simulink model "Inverse_Dynamic_Control"  (R2023b)
settings: Solver=FixedStepAuto  StartTime=0.0  StopTime=10.0  FixedStep=sampleTime  RelTol=1e-3
undefined symbols (not defined in the file): initial, initialPos, robot
libraries: robotmaniplib x5, robotcorelib x2
settings Model: Creator=jake9  LastModifiedBy=jake9

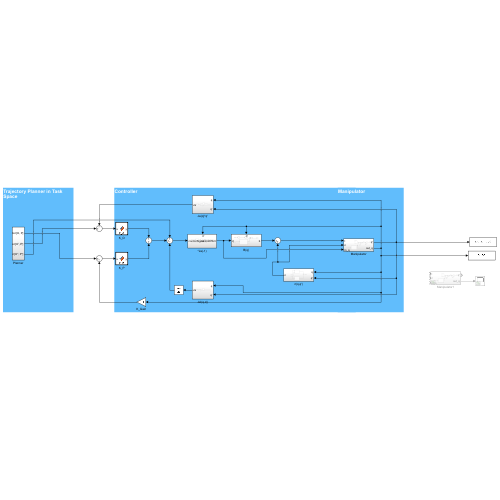
[thumbnail: Simulink's stored preview of the top-level diagram]
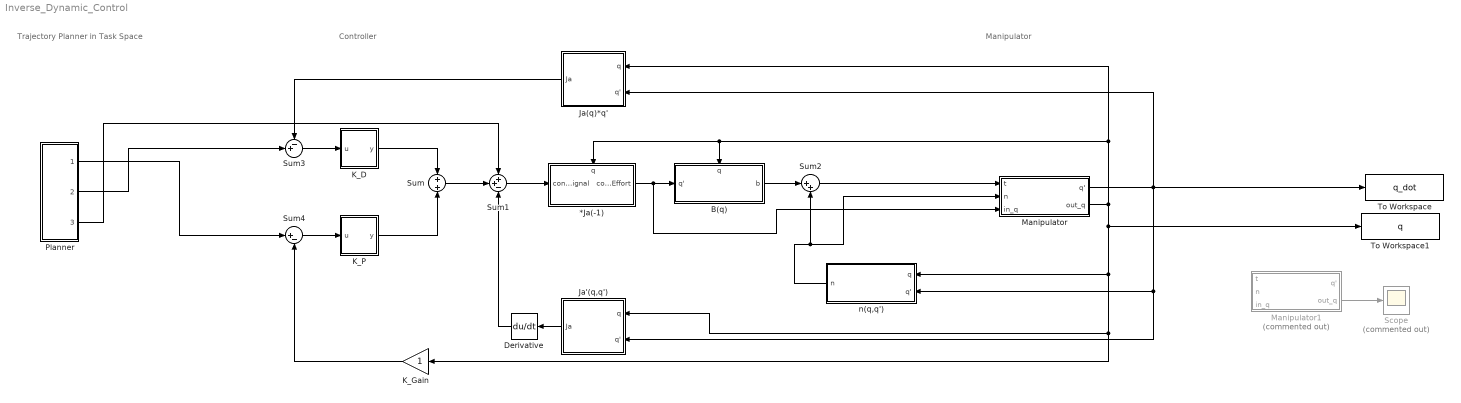
== system Inverse_Dynamic_Control ==
  note: Manipulator
  note: Trajectory Planner in Task Space
  note: Controller
  *Ja(-1) : Subsystem
      settings: PortSchema="{\"entries\":[{\"content\":{\"sides\":[{\"content\":{\"connectorIds\":[\"In1\"]},\"type\":\"ConnectorPlacement.EquallySpacedRectSide\",\"uuid\":\"6181597d-d95a-4c94-8b0a-1b126e10fdbf\"},{\"content\":{\"connectorIds\":[\"Out1\"],\"side\":\"RIGHT\"},\"type\":\"ConnectorPlacement.EquallySpacedRectSide\",\"uuid\":\"10cd4102-ac71-40d2-b2d5-351b2662a651\"},{\"content\":{\"connectorIds\":[\"In2\"],\"side\":\"TOP\"},\"type\":\"ConnectorPlacement.EquallySpacedRectSide\",\"uuid\":\"51fc8434-6bfd-4c46-b058-3c914862beda\"}]},\"type\":\"ConnectorPlacement.EquallySpacedConnector\",\"uuid\":\"e6979264-e48a-4d32-b7c0-5cbd3e80f60c\"}],\"packageUris\":[\"http://schema.mathworks.com/mf0/Connector/R2020b\"],\"version\":\"1.0\"}"
  B(q) : Subsystem
      settings: PortSchema="{\"entries\":[{\"content\":{\"sides\":[{\"content\":{\"connectorIds\":[\"In1\"]},\"type\":\"ConnectorPlacement.EquallySpacedRectSide\",\"uuid\":\"6181597d-d95a-4c94-8b0a-1b126e10fdbf\"},{\"content\":{\"connectorIds\":[\"Out1\"],\"side\":\"RIGHT\"},\"type\":\"ConnectorPlacement.EquallySpacedRectSide\",\"uuid\":\"10cd4102-ac71-40d2-b2d5-351b2662a651\"},{\"content\":{\"connectorIds\":[\"In2\"],\"side\":\"TOP\"},\"type\":\"ConnectorPlacement.EquallySpacedRectSide\",\"uuid\":\"51fc8434-6bfd-4c46-b058-3c914862beda\"}]},\"type\":\"ConnectorPlacement.EquallySpacedConnector\",\"uuid\":\"e6979264-e48a-4d32-b7c0-5cbd3e80f60c\"}],\"packageUris\":[\"http://schema.mathworks.com/mf0/Connector/R2020b\"],\"version\":\"1.0\"}"
  Derivative : Derivative
  Ja'(q,q') : Subsystem
  Ja(q)*q' : Subsystem
  K_D : MATLAB Function  TreatAsAtomicUnit=on
  K_Gain : Gain
  K_P : MATLAB Function  TreatAsAtomicUnit=on
  Manipulator : Subsystem
  Manipulator1 : Subsystem  Commented=on
  Planner : Subsystem
  Scope : Scope  Commented=on
  Sum : Sum  Inputs=+|+
  Sum1 : Sum  Inputs=++-
  Sum2 : Sum  Inputs=|++
  Sum3 : Sum  Inputs=-+|
  Sum4 : Sum  Inputs=|+-
  To Workspace : ToWorkspace  VariableName=q_dot  SampleTime=-1
  To Workspace1 : ToWorkspace  VariableName=q  SampleTime=-1
  n(q,q') : Subsystem
  wires:
  K_D/1(y) -> Sum/1
  K_P/1(y) -> Sum/2
  Sum/1 -> Sum1/2
  Sum1/1 -> *Ja(-1)/1(controlSignal)
  *Ja(-1)/1(controlEffort) -> Manipulator/3(in_q), B(q)/1(q')
  B(q)/1(b) -> Sum2/1
  Sum3/1 -> K_D/1(u)
  Sum4/1 -> K_P/1(u)
  K_Gain/1 -> Sum4/2
  n(q,q')/1(n) -> Manipulator/2(n), Sum2/2
  Sum2/1 -> Manipulator/1(t)
  Manipulator/2(out_q) -> Ja(q)*q'/1(q), *Ja(-1)/2(q), B(q)/2(q), To Workspace1/1, n(q,q')/1(q), Ja'(q,q')/1(q), K_Gain/1
  Manipulator/1(q') -> n(q,q')/2(q'), Ja'(q,q')/2(q'), Ja(q)*q'/2(q'), To Workspace/1
  Ja(q)*q'/1(Ja) -> Sum3/1
  Ja'(q,q')/1(Ja) -> Derivative/1
  Derivative/1 -> Sum1/3
  Planner/1("Out [O, P]") -> Sum4/1
  Planner/2("Out [O', P']") -> Sum3/2
  Planner/3("Out [O'', P'']") -> Sum1/1
  Manipulator1/2(out_q) -> Scope/1

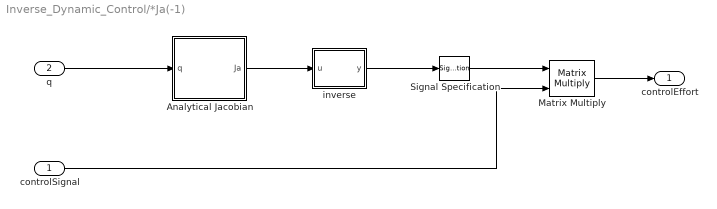
== system Inverse_Dynamic_Control/*Ja(-1) ==
  controlSignal : Inport
  q : Inport  Port=2
  Analytical Jacobian : Subsystem
  Matrix Multiply : Product  Multiplication=Matrix(*)
  Signal Specification : SignalSpecification  Dimensions=[6,6]
  inverse : MATLAB Function  TreatAsAtomicUnit=on
  controlEffort : Outport
  wires:
  q/1 -> Analytical Jacobian/1(q)
  controlSignal/1 -> Matrix Multiply/2
  inverse/1(y) -> Signal Specification/1
  Analytical Jacobian/1(Ja) -> inverse/1(u)
  Matrix Multiply/1 -> controlEffort/1
  Signal Specification/1 -> Matrix Multiply/1

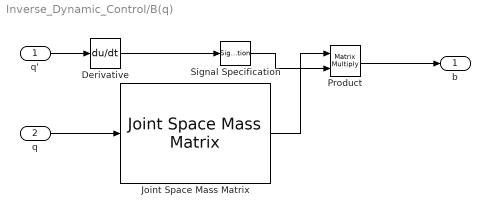
== system Inverse_Dynamic_Control/B(q) ==
  q' : Inport
  q : Inport  Port=2
  Derivative : Derivative
  Joint Space Mass Matrix : robotmaniplib/Joint Space Mass Matrix  RigidBodyTree=robot  SimulateUsing=Interpreted execution
  Product : Product  Multiplication=Matrix(*)
  Signal Specification : SignalSpecification  Dimensions=[6,1]
  b : Outport
  wires:
  q'/1 -> Derivative/1
  q/1 -> Joint Space Mass Matrix/1
  Product/1 -> b/1
  Derivative/1 -> Signal Specification/1
  Joint Space Mass Matrix/1 -> Product/1
  Signal Specification/1 -> Product/2

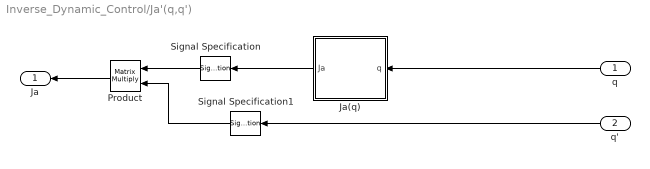
== system Inverse_Dynamic_Control/Ja'(q,q') ==
  q : Inport
  q' : Inport  Port=2
  Ja(q) : Subsystem
  Product : Product  Multiplication=Matrix(*)
  Signal Specification : SignalSpecification  Dimensions=[6,6]
  Signal Specification1 : SignalSpecification  Dimensions=[6,1]
  Ja : Outport
  wires:
  q/1 -> Ja(q)/1(q)
  q'/1 -> Signal Specification1/1
  Product/1 -> Ja/1
  Ja(q)/1(Ja) -> Signal Specification/1
  Signal Specification/1 -> Product/1
  Signal Specification1/1 -> Product/2

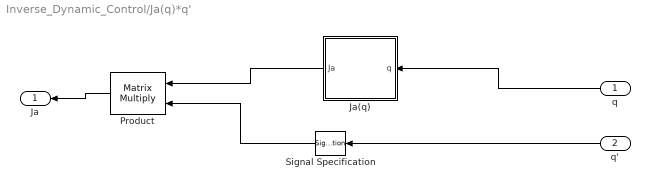
== system Inverse_Dynamic_Control/Ja(q)*q' ==
  q : Inport
  q' : Inport  Port=2
  Ja(q) : Subsystem
  Product : Product  Multiplication=Matrix(*)
  Signal Specification : SignalSpecification  Dimensions=[6,1]
  Ja : Outport
  wires:
  q/1 -> Ja(q)/1(q)
  Product/1 -> Ja/1
  Ja(q)/1(Ja) -> Product/1
  q'/1 -> Signal Specification/1
  Signal Specification/1 -> Product/2

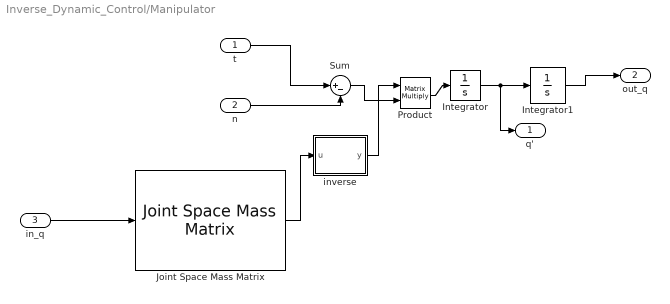
== system Inverse_Dynamic_Control/Manipulator ==
  t : Inport
  n : Inport  Port=2
  in_q : Inport  Port=3
  Integrator : Integrator  InitialCondition=initial
  Integrator1 : Integrator  InitialCondition=initialPos
  Joint Space Mass Matrix : robotmaniplib/Joint Space Mass Matrix  RigidBodyTree=robot  SimulateUsing=Interpreted execution
  Product : Product  Multiplication=Matrix(*)
  Sum : Sum  Inputs=|+-
  inverse : MATLAB Function  TreatAsAtomicUnit=on
  q' : Outport
  out_q : Outport  Port=2
  wires:
  Integrator/1 -> q'/1, Integrator1/1
  t/1 -> Sum/1
  n/1 -> Sum/2
  inverse/1(y) -> Product/1
  Sum/1 -> Product/2
  Product/1 -> Integrator/1
  Integrator1/1 -> out_q/1
  Joint Space Mass Matrix/1 -> inverse/1(u)
  in_q/1 -> Joint Space Mass Matrix/1

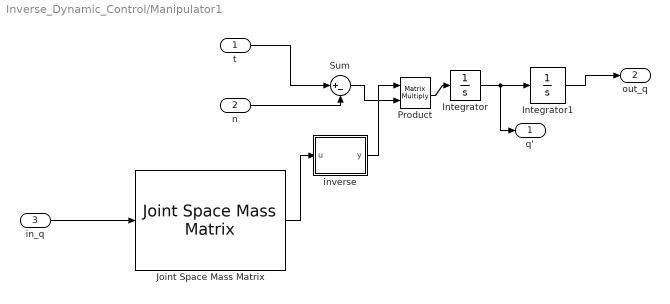
== system Inverse_Dynamic_Control/Manipulator1 ==
  t : Inport
  n : Inport  Port=2
  in_q : Inport  Port=3
  Integrator : Integrator  InitialCondition=initial
  Integrator1 : Integrator  InitialCondition=initialPos
  Joint Space Mass Matrix : robotmaniplib/Joint Space Mass Matrix  RigidBodyTree=robot  SimulateUsing=Interpreted execution
  Product : Product  Multiplication=Matrix(*)
  Sum : Sum  Inputs=|+-
  inverse : MATLAB Function  TreatAsAtomicUnit=on
  q' : Outport
  out_q : Outport  Port=2
  wires:
  Integrator/1 -> q'/1, Integrator1/1
  t/1 -> Sum/1
  n/1 -> Sum/2
  inverse/1(y) -> Product/1
  Sum/1 -> Product/2
  Product/1 -> Integrator/1
  Integrator1/1 -> out_q/1
  Joint Space Mass Matrix/1 -> inverse/1(u)
  in_q/1 -> Joint Space Mass Matrix/1

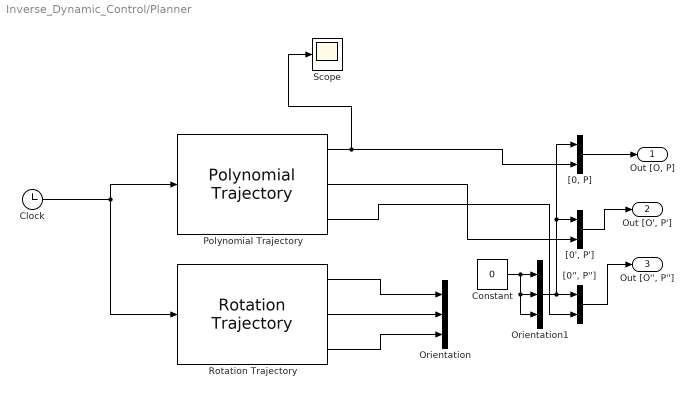
== system Inverse_Dynamic_Control/Planner ==
  Clock : Clock
  Constant : Constant  Value=0
  Orientation : Mux  Inputs=3
  Orientation1 : Mux  Inputs=3
  Polynomial Trajectory : robotcorelib/Polynomial Trajectory  WaypointSource=Internal  Waypoints=[1 1 1; 2 2 2; 3 3 3]'  TimePoints=[0, 4, 8]  TimeInterval=[ 1, 4 ]  Method=Cubic Polynomial  ParameterSource=Internal  VelocityBoundaryCondition=zeros( 3,3 )  AccelerationBoundaryCondition=zeros( 2, 5 )  SimulateUsing=Interpreted execution
  Rotation Trajectory : robotcorelib/Rotation Trajectory  WaypointFormat=Quaternion  WaypointSource=Internal  R0=[ 1, 0, 0, 0 ]'  RF=[ 0, 0, 1, 0 ]'  TimeInterval=[ 0, 8]  CustomTimeScaling=off  ParameterSource=Internal  TSTime=0:0.1:1  TimeScaling=[ 0:0.1:1; ones( 1, 11 ); zeros( 1, 11 ) ]  SimulateUsing=Interpreted execution
      settings: LibrarySourceBlock=robotutilslib/Rotation Trajectory
  Scope : Scope
  "[0'', P'']" : Mux  Inputs=2
  "[0', P']" : Mux  Inputs=2
  "[0, P]" : Mux  Inputs=2
  "Out [O, P]" : Outport
  "Out [O', P']" : Outport  Port=2
  "Out [O'', P'']" : Outport  Port=3
  wires:
  Clock/1 -> Rotation Trajectory/1, Polynomial Trajectory/1
  Polynomial Trajectory/1 -> "[0, P]"/2, Scope/1
  Polynomial Trajectory/2 -> "[0', P']"/2
  Polynomial Trajectory/3 -> "[0'', P'']"/2
  Rotation Trajectory/3 -> Orientation/3
  Rotation Trajectory/2 -> Orientation/2
  Rotation Trajectory/1 -> Orientation/1
  "[0, P]"/1 -> "Out [O, P]"/1
  Constant/1 -> Orientation1/3, Orientation1/2, Orientation1/1
  Orientation1/1 -> "[0'', P'']"/1, "[0', P']"/1, "[0, P]"/1
  "[0', P']"/1 -> "Out [O', P']"/1
  "[0'', P'']"/1 -> "Out [O'', P'']"/1

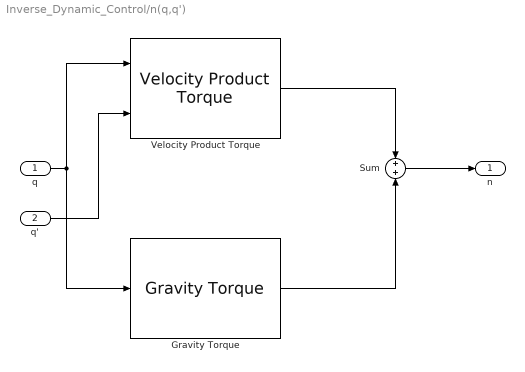
== system Inverse_Dynamic_Control/n(q,q') ==
  q : Inport
  q' : Inport  Port=2
  Gravity Torque : robotmaniplib/Gravity Torque  RigidBodyTree=robot  SimulateUsing=Interpreted execution
  Sum : Sum  Inputs=+|+
  Velocity Product Torque : robotmaniplib/Velocity Product Torque  RigidBodyTree=robot  SimulateUsing=Interpreted execution
  n : Outport
  wires:
  q/1 -> Gravity Torque/1, Velocity Product Torque/1
  q'/1 -> Velocity Product Torque/2
  Sum/1 -> n/1
  Gravity Torque/1 -> Sum/2
  Velocity Product Torque/1 -> Sum/1

== system Inverse_Dynamic_Control/*Ja(-1)/Analytical Jacobian ==
  note: Conversion of Jacobian, from Geometric to Analytical
      |
      | Matlab use the "Spatial Geometry" convenction, where the orientation in the first three rows instead of the last three rows. So we use:
      |
      | $J_{A}=\left[\begin{array}{cc} T^{-1} & 0 \\ 0 & I \end{array}\right]\left[\begin{array}{c} J_{O} \\ J_{P} \end{array}\right]=\left[\begin{array}{l} T^{-1} J_{O} \\ 0 \end{array}\right]+\left[\begin{array}{c} 0\\ J_{P} \end{array}\right] \quad \text {if } \,\, J=\left[\begin{array}{l} J_{O} \\ J_{P} \end{array}\right]$
      |
      | If orientation is in the last three rows (as in most of the text books) we would use instead:
      |
      | $J_{A}=\left[\begin{array}{cc} I & 0 \\ 0 & T^{-1} \end{array}\right]\left[\begin{array}{c} J_{P} \\ J_{O} \end{array}\right]=\left[\begin{array}{l} J_{P} \\ 0 \end{array}\right]+\left[\begin{array}{c} 0\\ T^{-1} J_{O} \end{array}\right] \quad \text { if } \,\, J=\left[\begin{array}{l} J_{P} \\ J_{O} \end{array}\right]$
  q : Inport
  Analytical from Geometric : MATLAB Function  TreatAsAtomicUnit=on
  Direct Kinematics : Subsystem
  Get Jacobian : Subsystem  mask(Get Jacobian){RigidBodyTree=robot, EndEffector=tool0, SimulateUsing=Code generation}
      mask prompts: RigidBodyTree "robotics:robotslmanip:blockmask:RigidBodyTreePrompt"; EndEffector "robotics:robotslmanip:blockmask:EndEffectorPrompt"; SimulateUsing "SystemBlock:MATLABSystem:SimulateUsing"
      mask help: robotics:robotslmanip:blockmask:GetJacobianDescription
      mask init:
      | try
      |    [TreeStruct, NumBodies, sysName] = robotics.slmanip.internal.block.RBTAlgorithmBlockMasks.updateMaskWorkSpaceVariables(gcb, RigidBodyTree);
      |    robotics.slmanip.internal.block.RBTAlgorithmBlockMasks.updateBlockInputDimensions(gcb, TreeStruct, 'Config');
      | catch ME
      |    TreeStruct = [];  NumBodies = [];   sysName = '???';
      |    throw(ME);
      | end
      | EndEffectorArray = robotics.slmanip.internal.block.RBTAlgorithmBlockMasks.updateBodyWSVar(gcb, RigidBodyTree, 'EndEffector');
      settings: LibrarySourceBlock=robotmaniplib/Get Jacobian
      mask Help: helpview(fullfile(docroot,'robotics','helptargets.map'), 'rstGetJacobian');
      mask TypeOptions SimulateUsing: MATLAB System/SimulateUsing
      mask DialogControl RigidBodyTree Prompt: Rigid body tree:
      mask DialogControl EndEffector Prompt: End effector:
      mask DialogControl ListControl Prompt: robotics:robotslmanip:blockmask:SelectBodyButtonPrompt
      mask DialogControl ListControl Callback: robotics.slmanip.internal.block.RBTAlgorithmBlockMasks.updateMaskBodyList(gcb, 'EndEffector');
      mask DialogControl SimulateUsing Prompt: Simulate using:
      mask DialogControl SimulateUsing Tooltip: SystemBlock:MATLABSystem:SimulateUsingDescription
      mask Display:
      | if (strcmp(sysName,'???'))
      | 	color('red');
      | else
      |     color('blue');
      | end
      | text(0.99, 0.99, sysName, 'horizontalAlignment', 'right', 'verticalAlignment','top');
      | 
      | color('black');
      | DescText = ['EE: ' get_param(gcb,'EndEffector')];
      | text(0.5, 0.05, DescText, 'horizontalAlignment', 'center', 'verticalAlignment','bottom');
      | 
      | port_label('input', 1, 'Config')
      | port_label('output', 1, 'Jacobian')
  Terminator : Terminator
  Ja : Outport
  wires:
  Direct Kinematics/1(orientation) -> Analytical from Geometric/2(angles)
  Direct Kinematics/2(position) -> Terminator/1
  Analytical from Geometric/1(Ja) -> Ja/1
  Get Jacobian/1(Jacobian) -> Analytical from Geometric/1(geomJ)
  q/1 -> Get Jacobian/1(Config), Direct Kinematics/1(q)

== system Inverse_Dynamic_Control/Ja'(q,q')/Ja(q) ==
  note: Conversion of Jacobian, from Geometric to Analytical
      |
      | Matlab use the "Spatial Geometry" convenction, where the orientation in the first three rows instead of the last three rows. So we use:
      |
      | $J_{A}=\left[\begin{array}{cc} T^{-1} & 0 \\ 0 & I \end{array}\right]\left[\begin{array}{c} J_{O} \\ J_{P} \end{array}\right]=\left[\begin{array}{l} T^{-1} J_{O} \\ 0 \end{array}\right]+\left[\begin{array}{c} 0\\ J_{P} \end{array}\right] \quad \text {if } \,\, J=\left[\begin{array}{l} J_{O} \\ J_{P} \end{array}\right]$
      |
      | If orientation is in the last three rows (as in most of the text books) we would use instead:
      |
      | $J_{A}=\left[\begin{array}{cc} I & 0 \\ 0 & T^{-1} \end{array}\right]\left[\begin{array}{c} J_{P} \\ J_{O} \end{array}\right]=\left[\begin{array}{l} J_{P} \\ 0 \end{array}\right]+\left[\begin{array}{c} 0\\ T^{-1} J_{O} \end{array}\right] \quad \text { if } \,\, J=\left[\begin{array}{l} J_{P} \\ J_{O} \end{array}\right]$
  q : Inport
  Analytical from Geometric : MATLAB Function  TreatAsAtomicUnit=on
  Direct Kinematics1 : Subsystem
  Get Jacobian : Subsystem  mask(Get Jacobian){RigidBodyTree=robot, EndEffector=tool0, SimulateUsing=Code generation}
      mask prompts: RigidBodyTree "robotics:robotslmanip:blockmask:RigidBodyTreePrompt"; EndEffector "robotics:robotslmanip:blockmask:EndEffectorPrompt"; SimulateUsing "SystemBlock:MATLABSystem:SimulateUsing"
      mask help: robotics:robotslmanip:blockmask:GetJacobianDescription
      mask init: same as Inverse_Dynamic_Control/*Ja(-1)/Analytical Jacobian/Get Jacobian
      settings: LibrarySourceBlock=robotmaniplib/Get Jacobian
      mask Help: helpview(fullfile(docroot,'robotics','helptargets.map'), 'rstGetJacobian');
      mask TypeOptions SimulateUsing: MATLAB System/SimulateUsing
      mask DialogControl RigidBodyTree Prompt: Rigid body tree:
      mask DialogControl EndEffector Prompt: End effector:
      mask DialogControl ListControl Prompt: robotics:robotslmanip:blockmask:SelectBodyButtonPrompt
      mask DialogControl ListControl Callback: robotics.slmanip.internal.block.RBTAlgorithmBlockMasks.updateMaskBodyList(gcb, 'EndEffector');
      mask DialogControl SimulateUsing Prompt: Simulate using:
      mask DialogControl SimulateUsing Tooltip: SystemBlock:MATLABSystem:SimulateUsingDescription
      mask Display:
      | if (strcmp(sysName,'???'))
      | 	color('red');
      | else
      |     color('blue');
      | end
      | text(0.99, 0.99, sysName, 'horizontalAlignment', 'right', 'verticalAlignment','top');
      | 
      | color('black');
      | DescText = ['EE: ' get_param(gcb,'EndEffector')];
      | text(0.5, 0.05, DescText, 'horizontalAlignment', 'center', 'verticalAlignment','bottom');
      | 
      | port_label('input', 1, 'Config')
      | port_label('output', 1, 'Jacobian')
  Terminator : Terminator
  Ja : Outport
  wires:
  Analytical from Geometric/1(Ja) -> Ja/1
  Get Jacobian/1(Jacobian) -> Analytical from Geometric/1(geomJ)
  q/1 -> Direct Kinematics1/1(q), Get Jacobian/1(Config)
  Direct Kinematics1/2(position) -> Terminator/1
  Direct Kinematics1/1(orientation) -> Analytical from Geometric/2(angles)

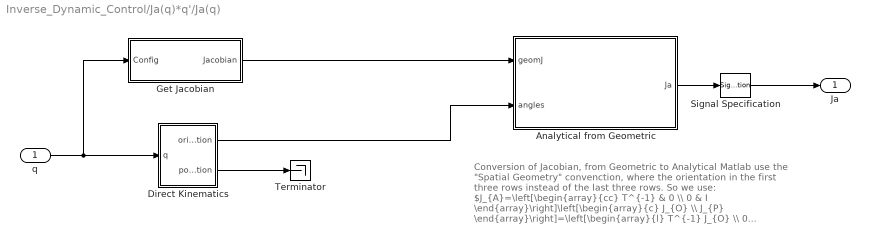
== system Inverse_Dynamic_Control/Ja(q)*q'/Ja(q) ==
  note: Conversion of Jacobian, from Geometric to Analytical
      |
      | Matlab use the "Spatial Geometry" convenction, where the orientation in the first three rows instead of the last three rows. So we use:
      |
      | $J_{A}=\left[\begin{array}{cc} T^{-1} & 0 \\ 0 & I \end{array}\right]\left[\begin{array}{c} J_{O} \\ J_{P} \end{array}\right]=\left[\begin{array}{l} T^{-1} J_{O} \\ 0 \end{array}\right]+\left[\begin{array}{c} 0\\ J_{P} \end{array}\right] \quad \text {if } \,\, J=\left[\begin{array}{l} J_{O} \\ J_{P} \end{array}\right]$
      |
      | If orientation is in the last three rows (as in most of the text books) we would use instead:
      |
      | $J_{A}=\left[\begin{array}{cc} I & 0 \\ 0 & T^{-1} \end{array}\right]\left[\begin{array}{c} J_{P} \\ J_{O} \end{array}\right]=\left[\begin{array}{l} J_{P} \\ 0 \end{array}\right]+\left[\begin{array}{c} 0\\ T^{-1} J_{O} \end{array}\right] \quad \text { if } \,\, J=\left[\begin{array}{l} J_{P} \\ J_{O} \end{array}\right]$
  q : Inport
  Analytical from Geometric : MATLAB Function  TreatAsAtomicUnit=on
  Direct Kinematics : Subsystem
  Get Jacobian : Subsystem  mask(Get Jacobian){RigidBodyTree=robot, EndEffector=tool0, SimulateUsing=Code generation}
      mask prompts: RigidBodyTree "robotics:robotslmanip:blockmask:RigidBodyTreePrompt"; EndEffector "robotics:robotslmanip:blockmask:EndEffectorPrompt"; SimulateUsing "SystemBlock:MATLABSystem:SimulateUsing"
      mask help: robotics:robotslmanip:blockmask:GetJacobianDescription
      mask init: same as Inverse_Dynamic_Control/*Ja(-1)/Analytical Jacobian/Get Jacobian
      settings: LibrarySourceBlock=robotmaniplib/Get Jacobian
      mask Help: helpview(fullfile(docroot,'robotics','helptargets.map'), 'rstGetJacobian');
      mask TypeOptions SimulateUsing: MATLAB System/SimulateUsing
      mask DialogControl RigidBodyTree Prompt: Rigid body tree:
      mask DialogControl EndEffector Prompt: End effector:
      mask DialogControl ListControl Prompt: robotics:robotslmanip:blockmask:SelectBodyButtonPrompt
      mask DialogControl ListControl Callback: robotics.slmanip.internal.block.RBTAlgorithmBlockMasks.updateMaskBodyList(gcb, 'EndEffector');
      mask DialogControl SimulateUsing Prompt: Simulate using:
      mask DialogControl SimulateUsing Tooltip: SystemBlock:MATLABSystem:SimulateUsingDescription
      mask Display:
      | if (strcmp(sysName,'???'))
      | 	color('red');
      | else
      |     color('blue');
      | end
      | text(0.99, 0.99, sysName, 'horizontalAlignment', 'right', 'verticalAlignment','top');
      | 
      | color('black');
      | DescText = ['EE: ' get_param(gcb,'EndEffector')];
      | text(0.5, 0.05, DescText, 'horizontalAlignment', 'center', 'verticalAlignment','bottom');
      | 
      | port_label('input', 1, 'Config')
      | port_label('output', 1, 'Jacobian')
  Signal Specification : SignalSpecification  Dimensions=[6,6]
  Terminator : Terminator
  Ja : Outport
  wires:
  Direct Kinematics/1(orientation) -> Analytical from Geometric/2(angles)
  Direct Kinematics/2(position) -> Terminator/1
  Analytical from Geometric/1(Ja) -> Signal Specification/1
  Get Jacobian/1(Jacobian) -> Analytical from Geometric/1(geomJ)
  q/1 -> Get Jacobian/1(Config), Direct Kinematics/1(q)
  Signal Specification/1 -> Ja/1

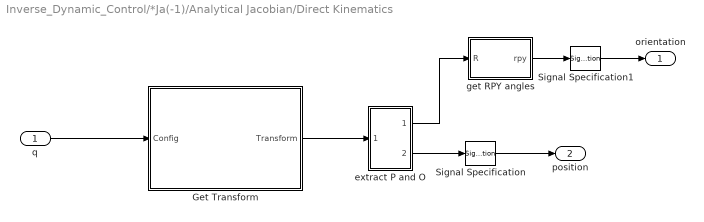
== system Inverse_Dynamic_Control/*Ja(-1)/Analytical Jacobian/Direct Kinematics ==
  q : Inport
  Get Transform : Subsystem  mask(Get Transform){RigidBodyTree=robot, SourceBody=tool0, TargetBody=base, SimulateUsing=Code generation}
      mask prompts: RigidBodyTree "robotics:robotslmanip:blockmask:RigidBodyTreePrompt"; SourceBody "robotics:robotslmanip:blockmask:GetTransformSourceBodyPrompt"; TargetBody "robotics:robotslmanip:blockmask:GetTransformTargetBodyPrompt"; SimulateUsing "SystemBlock:MATLABSystem:SimulateUsing"
      mask help: robotics:robotslmanip:blockmask:GetTransformDescription
      mask init:
      | try
      |    [TreeStruct, NumBodies, sysName] = robotics.slmanip.internal.block.RBTAlgorithmBlockMasks.updateMaskWorkSpaceVariables(gcb, RigidBodyTree);
      |    robotics.slmanip.internal.block.RBTAlgorithmBlockMasks.updateBlockInputDimensions(gcb, TreeStruct, 'Config');
      | catch ME
      |    TreeStruct = [];  NumBodies = [];   sysName = '???';
      |    throw(ME);
      | end
      | SourceBodyArray = robotics.slmanip.internal.block.RBTAlgorithmBlockMasks.updateBodyWSVar(gcb, RigidBodyTree, 'SourceBody');
      | TargetBodyArray = robotics.slmanip.internal.block.RBTAlgorithmBlockMasks.updateBodyWSVar(gcb, RigidBodyTree, 'TargetBody');
      settings: LibrarySourceBlock=robotmaniplib/Get Transform
      mask Help: helpview(fullfile(docroot,'robotics','helptargets.map'), 'rstGetTransform');
      mask TypeOptions SimulateUsing: MATLAB System/SimulateUsing
      mask DialogControl RigidBodyTree Prompt: Rigid body tree:
      mask DialogControl SourceBody Prompt: Source body:
      mask DialogControl ListControl1 Prompt: Select body >>
      mask DialogControl ListControl1 Callback: robotics.slmanip.internal.block.RBTAlgorithmBlockMasks.updateMaskBodyList(gcb, 'SourceBody');
      mask DialogControl TargetBody Prompt: Target body:
      mask DialogControl ListControl2 Prompt: Select body >>
      mask DialogControl ListControl2 Callback: robotics.slmanip.internal.block.RBTAlgorithmBlockMasks.updateMaskBodyList(gcb, 'TargetBody');
      mask DialogControl SimulateUsing Prompt: Simulate using:
      mask DialogControl SimulateUsing Tooltip: SystemBlock:MATLABSystem:SimulateUsingDescription
      mask Display:
      | if (strcmp(sysName,'???'))
      | 	color('red');
      | else
      |     color('blue');
      | end
      | text(0.99, 0.99, sysName, 'horizontalAlignment', 'right', 'verticalAlignment','top');
      | 
      | color('black')
      | SourceText = ['Source: ' get_param(gcb,'SourceBody')];
      | TargetText = ['Target: ' get_param(gcb,'TargetBody')];
      | DescText = [SourceText newline TargetText];
      | text(0.5, 0.05, DescText, 'horizontalAlignment', 'center','verticalAlignment','bottom');
      | 
      | port_label('input', 1, 'Config')
      | port_label('output', 1, 'Transform')
  Signal Specification : SignalSpecification  Dimensions=[3,1]
  Signal Specification1 : SignalSpecification  Dimensions=[3,1]
  extract P and O : Subsystem
  get RPY angles : MATLAB Function  TreatAsAtomicUnit=on
  orientation : Outport
  position : Outport  Port=2
  wires:
  extract P and O/1(orientation) -> get RPY angles/1(R)
  extract P and O/2(position) -> Signal Specification/1
  Get Transform/1(Transform) -> extract P and O/1(In1)
  q/1 -> Get Transform/1(Config)
  get RPY angles/1(rpy) -> Signal Specification1/1
  Signal Specification/1 -> position/1
  Signal Specification1/1 -> orientation/1

== system Inverse_Dynamic_Control/*Ja(-1)/Analytical Jacobian/Get Jacobian ==
  Config : Inport  PortDimensions=6
  MATLAB System : MATLABSystem  System=robotics.slmanip.internal.block.GetJacobianBlock  TreeStruct=TreeStruct  EEBodyName=EndEffector  SimulateUsing=Code generation
      mask Type: robotics.slmanip.internal.block.GetJacobianBlock
      mask Display:
      | disp('GetJacobianBlock');
      | port_label('input',1,'q');
      | port_label('output',1,'jacobianMat');
  Jacobian : Outport  VectorParamsAs1DForOutWhenUnconnected=off
  wires:
  MATLAB System/1 -> Jacobian/1
  Config/1 -> MATLAB System/1

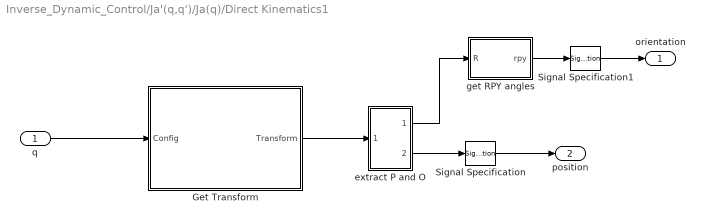
== system Inverse_Dynamic_Control/Ja'(q,q')/Ja(q)/Direct Kinematics1 ==
  q : Inport
  Get Transform : Subsystem  mask(Get Transform){RigidBodyTree=robot, SourceBody=tool0, TargetBody=base, SimulateUsing=Code generation}
      mask prompts: RigidBodyTree "robotics:robotslmanip:blockmask:RigidBodyTreePrompt"; SourceBody "robotics:robotslmanip:blockmask:GetTransformSourceBodyPrompt"; TargetBody "robotics:robotslmanip:blockmask:GetTransformTargetBodyPrompt"; SimulateUsing "SystemBlock:MATLABSystem:SimulateUsing"
      mask help: robotics:robotslmanip:blockmask:GetTransformDescription
      mask init: same as Inverse_Dynamic_Control/*Ja(-1)/Analytical Jacobian/Direct Kinematics/Get Transform
      settings: LibrarySourceBlock=robotmaniplib/Get Transform
      mask Help: helpview(fullfile(docroot,'robotics','helptargets.map'), 'rstGetTransform');
      mask TypeOptions SimulateUsing: MATLAB System/SimulateUsing
      mask DialogControl RigidBodyTree Prompt: Rigid body tree:
      mask DialogControl SourceBody Prompt: Source body:
      mask DialogControl ListControl1 Prompt: Select body >>
      mask DialogControl ListControl1 Callback: robotics.slmanip.internal.block.RBTAlgorithmBlockMasks.updateMaskBodyList(gcb, 'SourceBody');
      mask DialogControl TargetBody Prompt: Target body:
      mask DialogControl ListControl2 Prompt: Select body >>
      mask DialogControl ListControl2 Callback: robotics.slmanip.internal.block.RBTAlgorithmBlockMasks.updateMaskBodyList(gcb, 'TargetBody');
      mask DialogControl SimulateUsing Prompt: Simulate using:
      mask DialogControl SimulateUsing Tooltip: SystemBlock:MATLABSystem:SimulateUsingDescription
      mask Display:
      | if (strcmp(sysName,'???'))
      | 	color('red');
      | else
      |     color('blue');
      | end
      | text(0.99, 0.99, sysName, 'horizontalAlignment', 'right', 'verticalAlignment','top');
      | 
      | color('black')
      | SourceText = ['Source: ' get_param(gcb,'SourceBody')];
      | TargetText = ['Target: ' get_param(gcb,'TargetBody')];
      | DescText = [SourceText newline TargetText];
      | text(0.5, 0.05, DescText, 'horizontalAlignment', 'center','verticalAlignment','bottom');
      | 
      | port_label('input', 1, 'Config')
      | port_label('output', 1, 'Transform')
  Signal Specification : SignalSpecification  Dimensions=[3,1]
  Signal Specification1 : SignalSpecification  Dimensions=[3,1]
  extract P and O : Subsystem
  get RPY angles : MATLAB Function  TreatAsAtomicUnit=on
  orientation : Outport
  position : Outport  Port=2
  wires:
  extract P and O/1(orientation) -> get RPY angles/1(R)
  extract P and O/2(position) -> Signal Specification/1
  Get Transform/1(Transform) -> extract P and O/1(In1)
  q/1 -> Get Transform/1(Config)
  get RPY angles/1(rpy) -> Signal Specification1/1
  Signal Specification/1 -> position/1
  Signal Specification1/1 -> orientation/1

== system Inverse_Dynamic_Control/Ja'(q,q')/Ja(q)/Get Jacobian ==
  Config : Inport  PortDimensions=6
  MATLAB System : MATLABSystem  System=robotics.slmanip.internal.block.GetJacobianBlock  TreeStruct=TreeStruct  EEBodyName=EndEffector  SimulateUsing=Code generation
      mask Type: robotics.slmanip.internal.block.GetJacobianBlock
      mask Display:
      | disp('GetJacobianBlock');
      | port_label('input',1,'q');
      | port_label('output',1,'jacobianMat');
  Jacobian : Outport  VectorParamsAs1DForOutWhenUnconnected=off
  wires:
  MATLAB System/1 -> Jacobian/1
  Config/1 -> MATLAB System/1

== system Inverse_Dynamic_Control/Ja(q)*q'/Ja(q)/Direct Kinematics ==
  q : Inport
  Get Transform : Subsystem  mask(Get Transform){RigidBodyTree=robot, SourceBody=tool0, TargetBody=base, SimulateUsing=Code generation}
      mask prompts: RigidBodyTree "robotics:robotslmanip:blockmask:RigidBodyTreePrompt"; SourceBody "robotics:robotslmanip:blockmask:GetTransformSourceBodyPrompt"; TargetBody "robotics:robotslmanip:blockmask:GetTransformTargetBodyPrompt"; SimulateUsing "SystemBlock:MATLABSystem:SimulateUsing"
      mask help: robotics:robotslmanip:blockmask:GetTransformDescription
      mask init: same as Inverse_Dynamic_Control/*Ja(-1)/Analytical Jacobian/Direct Kinematics/Get Transform
      settings: LibrarySourceBlock=robotmaniplib/Get Transform
      mask Help: helpview(fullfile(docroot,'robotics','helptargets.map'), 'rstGetTransform');
      mask TypeOptions SimulateUsing: MATLAB System/SimulateUsing
      mask DialogControl RigidBodyTree Prompt: Rigid body tree:
      mask DialogControl SourceBody Prompt: Source body:
      mask DialogControl ListControl1 Prompt: Select body >>
      mask DialogControl ListControl1 Callback: robotics.slmanip.internal.block.RBTAlgorithmBlockMasks.updateMaskBodyList(gcb, 'SourceBody');
      mask DialogControl TargetBody Prompt: Target body:
      mask DialogControl ListControl2 Prompt: Select body >>
      mask DialogControl ListControl2 Callback: robotics.slmanip.internal.block.RBTAlgorithmBlockMasks.updateMaskBodyList(gcb, 'TargetBody');
      mask DialogControl SimulateUsing Prompt: Simulate using:
      mask DialogControl SimulateUsing Tooltip: SystemBlock:MATLABSystem:SimulateUsingDescription
      mask Display:
      | if (strcmp(sysName,'???'))
      | 	color('red');
      | else
      |     color('blue');
      | end
      | text(0.99, 0.99, sysName, 'horizontalAlignment', 'right', 'verticalAlignment','top');
      | 
      | color('black')
      | SourceText = ['Source: ' get_param(gcb,'SourceBody')];
      | TargetText = ['Target: ' get_param(gcb,'TargetBody')];
      | DescText = [SourceText newline TargetText];
      | text(0.5, 0.05, DescText, 'horizontalAlignment', 'center','verticalAlignment','bottom');
      | 
      | port_label('input', 1, 'Config')
      | port_label('output', 1, 'Transform')
  extract P and O : Subsystem
  get RPY angles : MATLAB Function  TreatAsAtomicUnit=on
  orientation : Outport
  position : Outport  Port=2
  wires:
  get RPY angles/1(rpy) -> orientation/1
  extract P and O/1(orientation) -> get RPY angles/1(R)
  extract P and O/2(position) -> position/1
  Get Transform/1(Transform) -> extract P and O/1(In1)
  q/1 -> Get Transform/1(Config)

== system Inverse_Dynamic_Control/Ja(q)*q'/Ja(q)/Get Jacobian ==
  Config : Inport  PortDimensions=6
  MATLAB System : MATLABSystem  System=robotics.slmanip.internal.block.GetJacobianBlock  TreeStruct=TreeStruct  EEBodyName=EndEffector  SimulateUsing=Code generation
      mask Type: robotics.slmanip.internal.block.GetJacobianBlock
      mask Display:
      | disp('GetJacobianBlock');
      | port_label('input',1,'q');
      | port_label('output',1,'jacobianMat');
  Jacobian : Outport  VectorParamsAs1DForOutWhenUnconnected=off
  wires:
  MATLAB System/1 -> Jacobian/1
  Config/1 -> MATLAB System/1

== system Inverse_Dynamic_Control/*Ja(-1)/Analytical Jacobian/Direct Kinematics/Get Transform ==
  Config : Inport  PortDimensions=6
  MATLAB System : MATLABSystem  System=robotics.slmanip.internal.block.GetTransformBlock  TreeStruct=TreeStruct  SourceBodyName=SourceBody  TargetBodyName=TargetBody  SimulateUsing=Code generation
      mask Type: robotics.slmanip.internal.block.GetTransformBlock
      mask Display:
      | disp('GetTransformBlock');
      | port_label('input',1,'q');
      | port_label('output',1,'tform');
  Transform : Outport  VectorParamsAs1DForOutWhenUnconnected=off
  wires:
  MATLAB System/1 -> Transform/1
  Config/1 -> MATLAB System/1

== system Inverse_Dynamic_Control/*Ja(-1)/Analytical Jacobian/Direct Kinematics/extract P and O ==
  In1 : Inport
  Orientation : MATLABFcn  MATLABFcn=tform2rotm  Output1D=off
  Position : MATLABFcn  MATLABFcn=tform2trvec
  orientation : Outport
  position : Outport  Port=2
  wires:
  Orientation/1 -> orientation/1
  In1/1 -> Position/1, Orientation/1
  Position/1 -> position/1

== system Inverse_Dynamic_Control/Ja'(q,q')/Ja(q)/Direct Kinematics1/Get Transform ==
  Config : Inport  PortDimensions=6
  MATLAB System : MATLABSystem  System=robotics.slmanip.internal.block.GetTransformBlock  TreeStruct=TreeStruct  SourceBodyName=SourceBody  TargetBodyName=TargetBody  SimulateUsing=Code generation
      mask Type: robotics.slmanip.internal.block.GetTransformBlock
      mask Display:
      | disp('GetTransformBlock');
      | port_label('input',1,'q');
      | port_label('output',1,'tform');
  Transform : Outport  VectorParamsAs1DForOutWhenUnconnected=off
  wires:
  MATLAB System/1 -> Transform/1
  Config/1 -> MATLAB System/1

== system Inverse_Dynamic_Control/Ja'(q,q')/Ja(q)/Direct Kinematics1/extract P and O ==
  In1 : Inport
  Orientation : MATLABFcn  MATLABFcn=tform2rotm  Output1D=off
  Position : MATLABFcn  MATLABFcn=tform2trvec
  orientation : Outport
  position : Outport  Port=2
  wires:
  Orientation/1 -> orientation/1
  In1/1 -> Position/1, Orientation/1
  Position/1 -> position/1

== system Inverse_Dynamic_Control/Ja(q)*q'/Ja(q)/Direct Kinematics/Get Transform ==
  Config : Inport  PortDimensions=6
  MATLAB System : MATLABSystem  System=robotics.slmanip.internal.block.GetTransformBlock  TreeStruct=TreeStruct  SourceBodyName=SourceBody  TargetBodyName=TargetBody  SimulateUsing=Code generation
      mask Type: robotics.slmanip.internal.block.GetTransformBlock
      mask Display:
      | disp('GetTransformBlock');
      | port_label('input',1,'q');
      | port_label('output',1,'tform');
  Transform : Outport  VectorParamsAs1DForOutWhenUnconnected=off
  wires:
  MATLAB System/1 -> Transform/1
  Config/1 -> MATLAB System/1

== system Inverse_Dynamic_Control/Ja(q)*q'/Ja(q)/Direct Kinematics/extract P and O ==
  In1 : Inport
  Orientation : MATLABFcn  MATLABFcn=tform2rotm  Output1D=off
  Position : MATLABFcn  MATLABFcn=tform2trvec
  orientation : Outport
  position : Outport  Port=2
  wires:
  Orientation/1 -> orientation/1
  In1/1 -> Position/1, Orientation/1
  Position/1 -> position/1

== matlab function Inverse_Dynamic_Control/*Ja(-1)/inverse ==
  data: u input; y output
function y = fcn(u)

y = inv(u);

== matlab function Inverse_Dynamic_Control/*Ja(-1)/Analytical Jacobian/Direct Kinematics/get RPY angles ==
  data: R input; rpy output
function rpy = rpyWrap(R)
%rpy = getRPYanglesFromR(R);
[rpy, ~] = eulerInverseProblem(R,'zyx','current');

== matlab function Inverse_Dynamic_Control/Ja(q)*q'/Ja(q)/Direct Kinematics/get RPY angles ==
  data: R input; rpy output
function rpy = rpyWrap(R)
%rpy = getRPYanglesFromR(R);
[rpy, ~] = eulerInverseProblem(R,'zyx','current');

== matlab function Inverse_Dynamic_Control/*Ja(-1)/Analytical Jacobian/Analytical from Geometric ==
  data: geomJ input; Ja output; angles input
function Ja = JacobAnFromGeomWrapper(geomJ,angles)
% For T^-1 matrix using RPY i.e., z(r) y(p) x(y) wrt to the current frame

T = rpy2Tmatrix(angles);

Tinv = inv(T);

% Following matlab convention (Jo is on top of Jp)
Ja = [Tinv,zeros(3);zeros(3),eye(3)] * geomJ;

% In standard convention one would have:
% analytJ = [eye(3),zeros(3);zeros(3),Tinv] * geomJ;

== matlab function Inverse_Dynamic_Control/Ja'(q,q')/Ja(q)/Analytical from Geometric ==
  data: geomJ input; Ja output; angles input
function Ja = JacobAnFromGeomWrapper(geomJ,angles)
% For T^-1 matrix using RPY i.e., z(r) y(p) x(y) wrt to the current frame

T = rpy2Tmatrix(angles);

Tinv = inv(T);

% Following matlab convention (Jo is on top of Jp)
Ja = [Tinv,zeros(3);zeros(3),eye(3)] * geomJ;

% In standard convention one would have:
% analytJ = [eye(3),zeros(3);zeros(3),Tinv] * geomJ;

== matlab function Inverse_Dynamic_Control/Manipulator/inverse ==
  data: u input; y output
function y = fcn(u)

y = inv(u);

== matlab function Inverse_Dynamic_Control/K_D ==
  data: u input; y output
function y = k_d(u)

kd = eye(6);
kd(4, 4) = 3;
kd(5, 5) = 3;
kd(6, 6) = 3;
y = kd * u;

== matlab function Inverse_Dynamic_Control/K_P ==
  data: u input; y output
function y = k_p(u)

kp = eye(6);
kp(4, 4) = 3;
kp(5, 5) = 3;
kp(6, 6) = 3;
y = kp * u;

== matlab function Inverse_Dynamic_Control/Ja'(q,q')/Ja(q)/Direct Kinematics1/get RPY angles ==
  data: R input; rpy output
function rpy = rpyWrap(R)
%rpy = getRPYanglesFromR(R);
[rpy, ~] = eulerInverseProblem(R,'zyx','current');

== matlab function Inverse_Dynamic_Control/Ja(q)*q'/Ja(q)/Analytical from Geometric ==
  data: geomJ input; Ja output; angles input
function Ja = JacobAnFromGeomWrapper(geomJ,angles)
% For T^-1 matrix using RPY i.e., z(r) y(p) x(y) wrt to the current frame

T = rpy2Tmatrix(angles);

Tinv = inv(T);

% Following matlab convention (Jo is on top of Jp)
Ja = [Tinv,zeros(3);zeros(3),eye(3)] * geomJ;

% In standard convention one would have:
% analytJ = [eye(3),zeros(3);zeros(3),Tinv] * geomJ;

== matlab function Inverse_Dynamic_Control/Manipulator1/inverse ==
  data: u input; y output
function y = fcn(u)

y = inv(u);
